simulink model "MBDq3"  (R2020a)
settings: Solver=VariableStepAuto  StartTime=0.0  StopTime=10.0  RelTol=1e-3
settings Model: Creator=DELL  LastModifiedBy=DELL

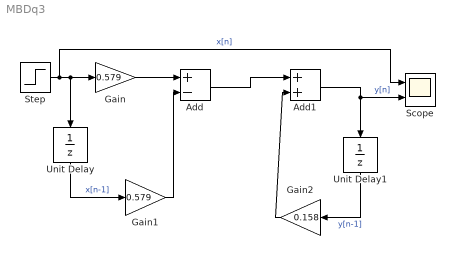
== system MBDq3 ==
  Add : Sum  Inputs=+-
  Add1 : Sum
  Gain : Gain  Gain=0.579
  Gain1 : Gain  Gain=0.579
  Gain2 : Gain  Gain=0.158
  Scope : Scope  NumInputPorts=2
  Step : Step  SampleTime=0
  Unit Delay : UnitDelay  SampleTime=-1  HasFrameUpgradeWarning=on
  Unit Delay1 : UnitDelay  SampleTime=-1  HasFrameUpgradeWarning=on
  wires:
  Step/1 -> Scope/1, Unit Delay/1, Gain/1  "x[n]"
  Unit Delay/1 -> Gain1/1  "x[n-1]"
  Gain1/1 -> Add/2
  Gain/1 -> Add/1
  Add/1 -> Add1/1
  Add1/1 -> Unit Delay1/1, Scope/2  "y[n]"
  Unit Delay1/1 -> Gain2/1  "y[n-1]"
  Gain2/1 -> Add1/2
